simulink model "SF045A_HwAgSysArbn"  (R2013b)
settings: Solver=FixedStepDiscrete  SolverMode=SingleTasking  StartTime=0.0  StopTime=1  FixedStep=.002  RelTol=1e-3
values from neighbouring files (symbols this model uses):
  ARCHGLBPRM_2MILLISEC_SEC_F32 = DataDict.Constant    [SF045A_HwAgSysArbn_DataDict.m]
  CNVSECTOCNT_CNTPERSEC_U32 = DataDict.Constant    [SF045A_HwAgSysArbn_DataDict.m]
  CNVTOMILLISEC_MILLISECPERCNT_F32 = DataDict.Constant    [SF045A_HwAgSysArbn_DataDict.m]
  FltInj_f32 = DataDict.Client    [SF045A_HwAgSysArbn_DataDict.m]
  FLTINJ_HWAGSYSARBN_HWAG = DataDict.Constant    [SF045A_HwAgSysArbn_DataDict.m]
  FLTINJ_HWAGSYSARBN_SERLCOMHWAG = DataDict.Constant    [SF045A_HwAgSysArbn_DataDict.m]
  HwAgSysArbnHwAgConf1Snsr = DataDict.Calibration    [SF045A_HwAgSysArbn_DataDict.m]
  HwAgSysArbnHwAgConf2Snsr = DataDict.Calibration    [SF045A_HwAgSysArbn_DataDict.m]
  HwAgSysArbnHwAgConfNoSnsr = DataDict.Calibration    [SF045A_HwAgSysArbn_DataDict.m]
  HwAgSysArbnHwAgCorrdCorrlnThd = DataDict.Calibration    [SF045A_HwAgSysArbn_DataDict.m]
  HwAgSysArbnHwAgCorrlnFailDebStep = DataDict.Calibration    [SF045A_HwAgSysArbn_DataDict.m]
  HwAgSysArbnHwAgCorrlnPassDebStep = DataDict.Calibration    [SF045A_HwAgSysArbn_DataDict.m]
  HwAgSysArbnHwAgCorrlnRng = DataDict.Calibration    [SF045A_HwAgSysArbn_DataDict.m]
  HwAgSysArbnHwAgSlewRate = DataDict.Calibration    [SF045A_HwAgSysArbn_DataDict.m]
  HwAgSysArbnHwAgSnsrlsCorrlnThd = DataDict.Calibration    [SF045A_HwAgSysArbn_DataDict.m]
  HwAgSysArbnHwAgSnsrlsKineThd = DataDict.Calibration    [SF045A_HwAgSysArbn_DataDict.m]
  HwAgSysArbnHwAgToMotAgCorrlnElpdTiLim = DataDict.Calibration    [SF045A_HwAgSysArbn_DataDict.m]
  HwAgSysArbnSerlComHwAgCorrdConf = DataDict.Calibration    [SF045A_HwAgSysArbn_DataDict.m]
  HwAgSysArbnSerlComHwAgSnsrlsConf = DataDict.Calibration    [SF045A_HwAgSysArbn_DataDict.m]
  HwAgSysArbnSlewRateTmr = DataDict.Calibration    [SF045A_HwAgSysArbn_DataDict.m]
  HWAGTHD_ULS_FLOAT32 = DataDict.Constant    [SF045A_HwAgSysArbn_DataDict.m]
  INVLDSRC_CNT_S08 = DataDict.Constant    [SF045A_HwAgSysArbn_DataDict.m]
  LRGSLEW_HWDEGPERSEC_F32 = DataDict.Constant    [SF045A_HwAgSysArbn_DataDict.m]
  NODEBSTEP_CNT_U16 = DataDict.Constant    [SF045A_HwAgSysArbn_DataDict.m]
  SLEWINPROGS_CNT_LGC = DataDict.Constant    [SF045A_HwAgSysArbn_DataDict.m]
  SLEWNOTINPROGS_CNT_LGC = DataDict.Constant    [SF045A_HwAgSysArbn_DataDict.m]
  SNSRDATASRCSELD_CNT_S08 = DataDict.Constant    [SF045A_HwAgSysArbn_DataDict.m]
  SNSRLSDATASRCSELD_CNT_S08 = DataDict.Constant    [SF045A_HwAgSysArbn_DataDict.m]
  ZEROTMR_MILLISEC_F32 = DataDict.Constant    [SF045A_HwAgSysArbn_DataDict.m]
undefined symbols (not defined in the file or in its folder): NtcNr1, NtcSts1
libraries: simulink x10, NxtrLim x7, autosarlib x2, NxtrAbslt x2
(part 1 of 3)
settings Model: PauseTimes=0.48  CovFilter=UTP_SF045A_HwAgSysArbn_cov_flt_list  CovHTMLOptions=-sRT=1 -aTS=1 -bRG=1 -bTC=1 -hTR=0 -nFC=0 -scm=1 -bcm=1 -xEv=0  Creator=TZ5743  LastModifiedBy=TZ5743
settings SolverCC: AutoInsertRateTranBlk=on  InsertRTBMode=Always
settings DataIOCC: LimitDataPoints=off  SaveFormat=Structure  ReturnWorkspaceOutputs=on
settings OptimizationCC: BlockReduction=off  InlineParams=on  ZeroExternalMemoryAtStartup=off  ZeroInternalMemoryAtStartup=off  OptimizeModelRefInitCode=on  LifeSpan=1
settings DebuggingCC: SignalInfNanChecking=error  SignalRangeChecking=warning  UnderspecifiedInitializationDetection=Simplified  SolverPrmCheckMsg=error  InheritedTsInSrcMsg=error  DiscreteInheritContinuousMsg=error  SingleTaskRateTransMsg=error  TasksWithSamePriorityMsg=error  SigSpecEnsureSampleTimeMsg=error  CheckMatrixSingularityMsg=error  ParameterUnderflowMsg=error  ParameterPrecisionLossMsg=error  ParameterTunabilityLossMsg=error  FixptConstUnderflowMsg=warning  FixptConstOverflowMsg=warning  VectorMatrixConversionMsg=error  SignalLabelMismatchMsg=error  UnconnectedInputMsg=error  UnconnectedOutputMsg=error  UnconnectedLineMsg=error  SFcnCompatibilityMsg=error  UniqueDataStoreMsg=warning  BusObjectLabelMismatch=error  RootOutportRequireBusObject=error  AssertControl=DisableAll  ModelReferenceIOMsg=error  ModelReferenceVersionMismatchMessage=warning  ModelReferenceIOMismatchMessage=error  ModelReferenceCSMismatchMessage=warning  ModelReferenceDataLoggingMessage=error  StateNameClashWarn=warning  StrictBusMsg=ErrorOnBusTreatedAsVector  NonBusSignalsTreatedAsBus=error  SFUnexpectedBacktrackingDiag=error  SFInvalidInputDataAccessInChartInitDiag=error  SFNoUnconditionalDefaultTransitionDiag=error  SFTransitionOutsideNaturalParentDiag=error  SFUnconditionalTransitionShadowingDiag=error  SFUndirectedBroadcastEventsDiag=error
settings ModelReferenceCC: ModelReferenceNumInstancesAllowed=Single
settings RTWCC: SystemTargetFile=autosar.tlc  GenCodeOnly=on  TemplateMakefile=ert_default_tmf  Description=AUTOSAR  GenerateReport=on  ProcessScript=autosar_make_rtw_hook  LaunchReport=on
settings CodeAppCC: GenerateComments=off  IgnoreCustomStorageClasses=off  CustomSymbolStrType=$N$R$M  CustomSymbolStrBlkIO=$N$M  SimulinkBlockComments=off
settings STFCustomTargetCC: ParMdlRefBuildCompliant=on  CompOptLevelCompliant=on  IncludeMdlTerminateFcn=off  CombineOutputUpdateFcns=on  SuppressErrorStatus=on  ERTFirstTimeCompliant=on  ERTCustomFileBanners=on  SupportNonFinite=off  SupportComplex=off  SupportContinuousTime=off  SupportNonInlinedSFcns=off  MATLABClassNameForMDSCustomization=Simulink.SoftwareTarget.ERTCustomization  AutosarCompliant=on  GRTInterface=off  SystemTargetFile=autosar.tlc
settings ERTTargetCC: CodeReplacementLibrary=ANSI_C  ConcurrentExecutionCompliant=off  IncludeMdlTerminateFcn=off  SuppressErrorStatus=on  SupportNonFinite=off  SupportComplex=off  ModelStepFunctionPrototypeControlCompliant=off  CPPClassGenCompliant=off  AutosarCompliant=on  InlinedParameterPlacement=NonHierarchical  ERTCustomFileTemplate=example_file_process.tlc  EnableUserReplacementTypes=on

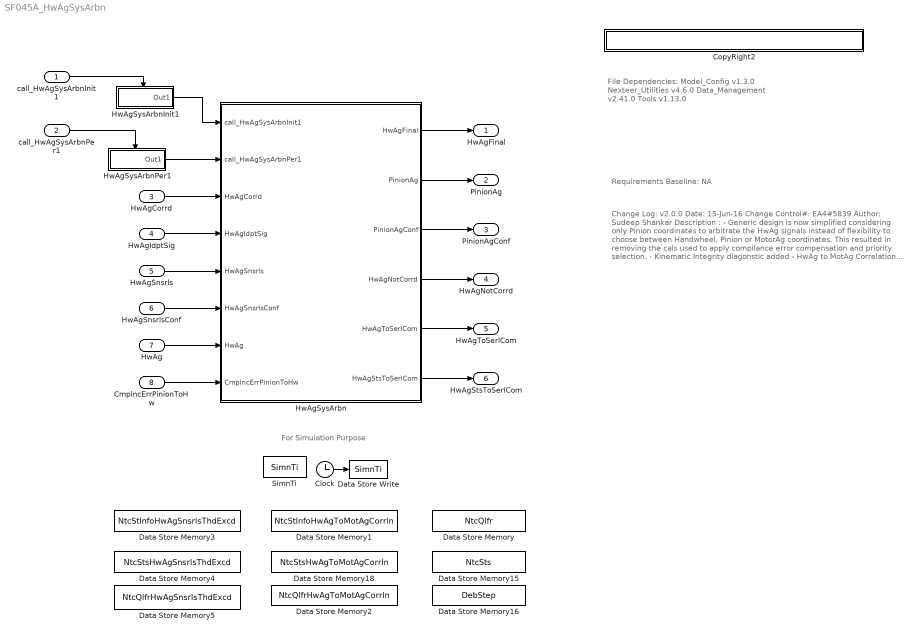
== system SF045A_HwAgSysArbn ==
  note: For Simulation Purpose
  note: File Dependencies:
      |
      | Model_Config v1.3.0
      | Nexteer_Utilities v4.6.0
      | Data_Management v2.41.0
      | Tools v1.13.0
  note: Requirements Baseline: NA
  note: Change Log:
      |
      | v2.0.0
      | Date: 15-Jun-16
      | Change Control#: EA4#5839
      | Author: Sudeep Shankar
      | Description :
      | - Generic design is now simplified considering only Pinion
      | coordinates to arbitrate the HwAg signals instead of flexibility to
      | choose between Handwheel, Pinion or MotorAg coordinates.
      | This resulted in removing the cals used to apply compilance error
      | compensation and priority selection.
      | - Kinematic Integrity diagonstic added
      | - HwAg to MotAg Correlation diagonstic added
      | - Logic added to arbitrate HwAg signal going to EOT when HwAg
      | sensor signals not available.
      |
      | v1.1.0
      | Date: 12-Sep-2015
      | Change Control #: EA4#860
      | Author:  Sudeep Shankar
      | Description:
      | - Minor modification in source change logic
      |  detection to avoid ambiguity in state variable
      |  read and write priorities
      | - Setting Initial condition of while loop to 'true'
      | instead of comparing greater than 1.
      | - Removed signal conversion blocks wherever
      | not required.
      | - Set while loop iteration to '-1' instead of restricting
      | it to '5' as condition check is in place to restrict
      | while iteration equal to number of signals present.
      |
      | v1.0.0
      | Date: 28-Aug-2015
      | Change Control #: EA4#860
      | Author:  Sudeep Shankar
      | Description:
      | - EA4 Initial Release
  call_HwAgSysArbnInit1 : Inport
  call_HwAgSysArbnPer1 : Inport  Port=2
  HwAgCorrd : Inport  RequirementInfo={} %GIDa_cc9a7bcf_75f9_45c8_a24f_b8479fae80cf  Port=3
  HwAgIdptSig : Inport  RequirementInfo={} %GIDa_9a7b919a_3c4b_44c1_bb96_545a47b8b3d3  Port=4
  HwAgSnsrls : Inport  RequirementInfo={} %GIDa_eede448f_64dd_4146_b16f_6fc16ca31f60  Port=5
  HwAgSnsrlsConf : Inport  RequirementInfo={} %GIDa_f6d9b3ed_9576_46cf_8319_2d07116884b2  Port=6
  HwAg : Inport  RequirementInfo={} %GIDa_3ab8439e_d791_45cf_9b38_dc1d6a5d96c4  Port=7
  CmplncErrPinionToHw : Inport  RequirementInfo={} %GIDa_8afc3a2b_29a0_4b25_ac8f_049b17fb3d6a  Port=8
  Clock : Clock
  CopyRight2 : Subsystem  Description=|  mask(Copyright Information){none=on}
      | Copyright info block.                                               
      |                                                                     
      | Place copyright information at the top of every subsystem in design.
      mask prompts: none "No parameters"
      mask help: Place copyright information at the top of every subsystem in design.
      mask Display:
      | NxtrConf = 'Nexteer Confidential';
      | 
      | sys = bdroot; %handle for the current model ("system")
      | first = get_param(sys,'Created');
      | first = first(end-3:end);  %year is last four digits
      | 
      | last = get_param(sys,'LastModifiedDate');
      | if isempty(last)
      |     last = datestr(now,'yyyy');
      | else
      |     last = last(end-3:end);
      | end
      | 
      | if strcmp(first,last)
      |     fprintf('%s -- Copyright %s Nexteer',NxtrConf,first)
      | else
      |     fprintf('%s -- %s%s- %s Nexteer',NxtrConf,char(169),first,last)
      | end
  Data Store Memory : DataStoreMemory  DataStoreName=NtcQlfr  InitialValue=SigQlfr1.SIGQLFR_NORES  OutDataTypeStr=Enum: SigQlfr1
  Data Store Memory1 : DataStoreMemory  DataStoreName=NtcStInfoHwAgToMotAgCorrln  OutDataTypeStr=uint8
  Data Store Memory15 : DataStoreMemory  DataStoreName=NtcSts  InitialValue=NtcSts1.NTCSTS_PREPASSD  OutDataTypeStr=Enum: NtcSts1
  Data Store Memory16 : DataStoreMemory  DataStoreName=DebStep
  Data Store Memory18 : DataStoreMemory  DataStoreName=NtcStsHwAgToMotAgCorrln  InitialValue=NtcSts1.NTCSTS_PASSD  OutDataTypeStr=Enum: NtcSts1
  Data Store Memory2 : DataStoreMemory  DataStoreName=NtcQlfrHwAgToMotAgCorrln  InitialValue=SigQlfr1.SIGQLFR_NORES  OutDataTypeStr=Enum: SigQlfr1
  Data Store Memory3 : DataStoreMemory  DataStoreName=NtcStInfoHwAgSnsrlsThdExcd  OutDataTypeStr=uint8
  Data Store Memory4 : DataStoreMemory  DataStoreName=NtcStsHwAgSnsrlsThdExcd  InitialValue=NtcSts1.NTCSTS_PASSD  OutDataTypeStr=Enum: NtcSts1
  Data Store Memory5 : DataStoreMemory  DataStoreName=NtcQlfrHwAgSnsrlsThdExcd  InitialValue=SigQlfr1.SIGQLFR_NORES  OutDataTypeStr=Enum: SigQlfr1
  Data Store Write : DataStoreWrite  DataStoreName=SimnTi
  HwAgSysArbn : Subsystem  RequirementInfo="{}  %GIDa_b3e0ed6f_fb94_4fa4_96b1_04061689a89e"
  HwAgSysArbnInit1 : Subsystem  TreatAsAtomicUnit=on
  HwAgSysArbnPer1 : Subsystem  TreatAsAtomicUnit=on
  SimnTi : DataStoreMemory  DataStoreName=SimnTi
  HwAgFinal : Outport
  PinionAg : Outport  Port=2
  PinionAgConf : Outport  Port=3
  HwAgNotCorrd : Outport  Port=4
  HwAgToSerlCom : Outport  Port=5
  HwAgStsToSerlCom : Outport  Port=6
  wires:
  HwAgSysArbn/2(PinionAg) -> PinionAg/1
  HwAgSysArbn/3(PinionAgConf) -> PinionAgConf/1
  HwAgSysArbn/4(HwAgNotCorrd) -> HwAgNotCorrd/1
  HwAgSysArbn/1(HwAgFinal) -> HwAgFinal/1
  HwAgSysArbn/6(HwAgStsToSerlCom) -> HwAgStsToSerlCom/1
  Clock/1 -> Data Store Write/1
  HwAgSysArbn/5(HwAgToSerlCom) -> HwAgToSerlCom/1
  HwAgSysArbnInit1/1(Out1) -> HwAgSysArbn/1(call_HwAgSysArbnInit1)
  HwAgSysArbnPer1/1(Out1) -> HwAgSysArbn/2(call_HwAgSysArbnPer1)
  HwAgSnsrls/1 -> HwAgSysArbn/5(HwAgSnsrls)
  HwAgCorrd/1 -> HwAgSysArbn/3(HwAgCorrd)
  HwAgSnsrlsConf/1 -> HwAgSysArbn/6(HwAgSnsrlsConf)
  HwAgIdptSig/1 -> HwAgSysArbn/4(HwAgIdptSig)
  CmplncErrPinionToHw/1 -> HwAgSysArbn/8(CmplncErrPinionToHw)
  HwAg/1 -> HwAgSysArbn/7(HwAg)
  call_HwAgSysArbnInit1/1 -> HwAgSysArbnInit1/Enable
  call_HwAgSysArbnPer1/1 -> HwAgSysArbnPer1/Enable

== system SF045A_HwAgSysArbn/CopyRight2 ==

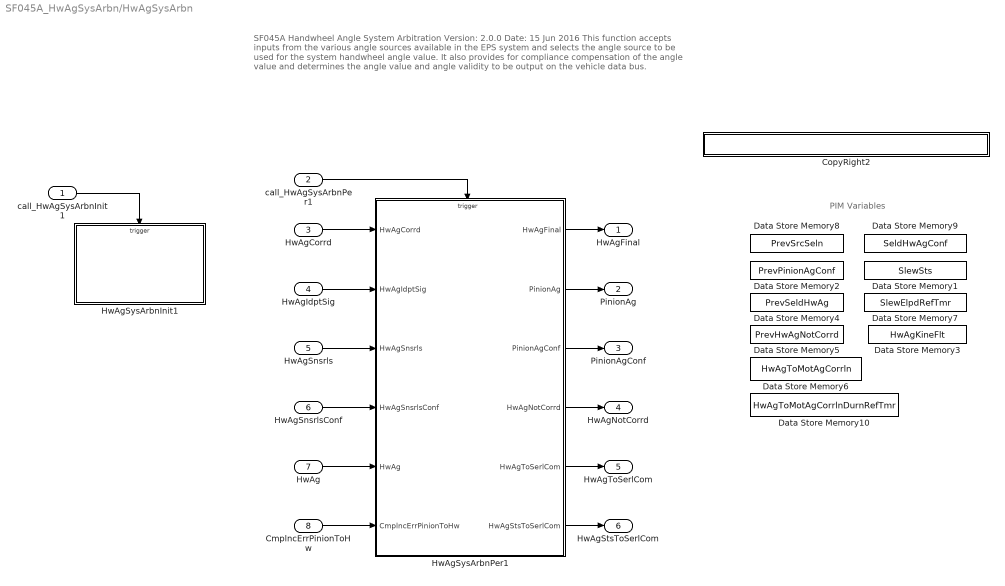
== system SF045A_HwAgSysArbn/HwAgSysArbn ==
  note: PIM Variables
  note: SF045A  Handwheel Angle System Arbitration       Version: 2.0.0                                                        Date: 15 Jun 2016
      |
      | This function accepts inputs from the various angle sources available in the EPS system and selects the angle
      | source to be used for the system handwheel angle value. It also provides for compliance compensation of the
      | angle value and determines the angle value and angle validity to be output on the vehicle data bus.
  call_HwAgSysArbnInit1 : Inport
  call_HwAgSysArbnPer1 : Inport  Port=2
  HwAgCorrd : Inport  RequirementInfo={} %GIDa_0c48395d_f55e_4aa8_967c_ddfcd5dc0f09  Port=3
  HwAgIdptSig : Inport  RequirementInfo={} %GIDa_050c3700_87b8_4e6a_a603_fe10bf5bb98d  Port=4
  HwAgSnsrls : Inport  RequirementInfo={} %GIDa_2af70a6d_5cf9_42e5_985f_0de67760f974  Port=5
  HwAgSnsrlsConf : Inport  RequirementInfo={} %GIDa_205f4441_a425_4e75_91eb_166c28519f31  Port=6
  HwAg : Inport  RequirementInfo={} %GIDa_bd860903_e40a_4856_a107_6e65debfd627  Port=7
  CmplncErrPinionToHw : Inport  RequirementInfo={} %GIDa_fd50d5ef_7c8c_43a4_8956_a275e6267051  Port=8
  CopyRight2 : Subsystem  Description=|  mask(Copyright Information){none=on}
      | Copyright info block.                                               
      |                                                                     
      | Place copyright information at the top of every subsystem in design.
      mask prompts: none "No parameters"
      mask help: Place copyright information at the top of every subsystem in design.
      mask Display:
      | NxtrConf = 'Nexteer Confidential';
      | 
      | sys = bdroot; %handle for the current model ("system")
      | first = get_param(sys,'Created');
      | first = first(end-3:end);  %year is last four digits
      | 
      | last = get_param(sys,'LastModifiedDate');
      | if isempty(last)
      |     last = datestr(now,'yyyy');
      | else
      |     last = last(end-3:end);
      | end
      | 
      | if strcmp(first,last)
      |     fprintf('%s -- Copyright %s Nexteer',NxtrConf,first)
      | else
      |     fprintf('%s -- %s%s- %s Nexteer',NxtrConf,char(169),first,last)
      | end
  Data Store Memory1 : DataStoreMemory  DataStoreName=SlewSts  StateMustResolveToSignalObject=on
  Data Store Memory10 : DataStoreMemory  DataStoreName=HwAgToMotAgCorrlnDurnRefTmr  StateMustResolveToSignalObject=on
  Data Store Memory2 : DataStoreMemory  DataStoreName=PrevPinionAgConf  StateMustResolveToSignalObject=on
  Data Store Memory3 : DataStoreMemory  DataStoreName=HwAgKineFlt  StateMustResolveToSignalObject=on
  Data Store Memory4 : DataStoreMemory  DataStoreName=PrevSeldHwAg  StateMustResolveToSignalObject=on
  Data Store Memory5 : DataStoreMemory  DataStoreName=PrevHwAgNotCorrd  StateMustResolveToSignalObject=on
  Data Store Memory6 : DataStoreMemory  DataStoreName=HwAgToMotAgCorrln  StateMustResolveToSignalObject=on
  Data Store Memory7 : DataStoreMemory  DataStoreName=SlewElpdRefTmr  StateMustResolveToSignalObject=on
  Data Store Memory8 : DataStoreMemory  DataStoreName=PrevSrcSeln  StateMustResolveToSignalObject=on
  Data Store Memory9 : DataStoreMemory  DataStoreName=SeldHwAgConf  StateMustResolveToSignalObject=on
  HwAgSysArbnInit1 : Subsystem  TreatAsAtomicUnit=on
  HwAgSysArbnPer1 : Subsystem
  HwAgFinal : Outport  RequirementInfo={} %GIDa_011fe0ec_bcc0_4a9e_bfa8_b93370ffdc5f
  PinionAg : Outport  RequirementInfo={} %GIDa_f176d339_cae7_40f0_af7d_2598900e3a6e  Port=2
  PinionAgConf : Outport  RequirementInfo={} %GIDa_ba6f2b72_e674_40ee_820e_69cfc9bdaacd  Port=3
  HwAgNotCorrd : Outport  RequirementInfo={} %GIDa_667dfd31_56c6_4848_b6a8_5a3d7a5632fb  Port=4
  HwAgToSerlCom : Outport  RequirementInfo={} %GIDa_8096249c_a6e2_4a31_b51a_c06af36d6bde  Port=5
  HwAgStsToSerlCom : Outport  RequirementInfo={} %GIDa_30b9e9dd_ad37_434a_8538_15d621b4541c  Port=6
  wires:
  call_HwAgSysArbnPer1/1 -> HwAgSysArbnPer1/Trigger
  call_HwAgSysArbnInit1/1 -> HwAgSysArbnInit1/Trigger
  HwAgSysArbnPer1/4(HwAgNotCorrd) -> HwAgNotCorrd/1
  HwAgSysArbnPer1/2(PinionAg) -> PinionAg/1
  HwAgSysArbnPer1/6(HwAgStsToSerlCom) -> HwAgStsToSerlCom/1
  HwAgSysArbnPer1/5(HwAgToSerlCom) -> HwAgToSerlCom/1
  HwAgSysArbnPer1/3(PinionAgConf) -> PinionAgConf/1
  HwAgSnsrls/1 -> HwAgSysArbnPer1/3(HwAgSnsrls)
  HwAgCorrd/1 -> HwAgSysArbnPer1/1(HwAgCorrd)
  HwAgSnsrlsConf/1 -> HwAgSysArbnPer1/4(HwAgSnsrlsConf)
  HwAgIdptSig/1 -> HwAgSysArbnPer1/2(HwAgIdptSig)
  CmplncErrPinionToHw/1 -> HwAgSysArbnPer1/6(CmplncErrPinionToHw)
  HwAg/1 -> HwAgSysArbnPer1/5(HwAg)
  HwAgSysArbnPer1/1(HwAgFinal) -> HwAgFinal/1

== system SF045A_HwAgSysArbn/HwAgSysArbnInit1 ==
  Enable : EnablePort
  Function-Call Generator : simulink/Ports & Subsystems/Function-Call Generator  sample_time=.002  numberOfIterations=1
  Out1 : Outport
  wires:
  Function-Call Generator/1 -> Out1/1

== system SF045A_HwAgSysArbn/HwAgSysArbnPer1 ==
  Enable : EnablePort
  call_HwAgSysArbnPer1 : simulink/Ports & Subsystems/Function-Call Generator  RequirementInfo={} %GIDa_ec825fb2_121b_4b6b_b290_bf31fce876d3  sample_time=0.002  numberOfIterations=1
  Out1 : Outport
  wires:
  call_HwAgSysArbnPer1/1 -> Out1/1

== system SF045A_HwAgSysArbn/HwAgSysArbn/CopyRight2 ==

== system SF045A_HwAgSysArbn/HwAgSysArbn/HwAgSysArbnInit1 ==
  note: Set Kinematic Integrity Diagostic to PASS
  note: 'PrevSrcSeln' is set to "INVALID SOURCE" in initialization to ensure that source change is detected
      | when source selection happens for the first time after initialization.
  note: Initialize Slew State to "Not in progress" at startup
  function : TriggerPort  TriggerType=function-call
  Constant1 : Constant  RequirementInfo={} %GIDa_bd6cf35a_c752_43ca_93be_9c9b276a6240  Value=0
  Constant2 : Constant  RequirementInfo={} %GIDa_50809f46_4379_44ea_9224_8e996deda18f  Value=NODEBSTEP_CNT_U16
  Constant7 : Constant  Value=SLEWNOTINPROGS_CNT_LGC
  CopyRight2 : Subsystem  Description=|  mask(Copyright Information){none=on}
      | Copyright info block.                                               
      |                                                                     
      | Place copyright information at the top of every subsystem in design.
      mask prompts: none "No parameters"
      mask help: Place copyright information at the top of every subsystem in design.
      mask Display:
      | NxtrConf = 'Nexteer Confidential';
      | 
      | sys = bdroot; %handle for the current model ("system")
      | first = get_param(sys,'Created');
      | first = first(end-3:end);  %year is last four digits
      | 
      | last = get_param(sys,'LastModifiedDate');
      | if isempty(last)
      |     last = datestr(now,'yyyy');
      | else
      |     last = last(end-3:end);
      | end
      | 
      | if strcmp(first,last)
      |     fprintf('%s -- Copyright %s Nexteer',NxtrConf,first)
      | else
      |     fprintf('%s -- %s%s- %s Nexteer',NxtrConf,char(169),first,last)
      | end
  Data Store Write1 : DataStoreWrite  RequirementInfo={} %GIDa_ed78b567_a6b6_41da_bf60_9df352ceaf90  DataStoreName=HwAgToMotAgCorrlnDurnRefTmr
  Data Store Write5 : DataStoreWrite  RequirementInfo={} %GIDa_5976233f_3450_4a81_8e0a_eaaf4d56a88e  DataStoreName=SlewSts
  Data Store Write6 : DataStoreWrite  RequirementInfo={} %GIDa_4cb2551e_dfbf_4575_8209_178b050baa05  DataStoreName=PrevSrcSeln
  Enumerated Constant1 : simulink/Sources/Enumerated Constant  RequirementInfo={} %GIDa_78dbafe2_a67d_4f00_b984_ee6afb604272  OutDataTypeStr=Enum: NtcSts1  Value=NtcSts1.NTCSTS_PASSD  SampleTime=inf
  Enumerated Constant2 : simulink/Sources/Enumerated Constant  RequirementInfo={} %GIDa_10ca5e51_019d_4f39_90cb_2775e488d2b0  OutDataTypeStr=Enum: NtcNr1  Value=NtcNr1.NTCNR_0X0A1  SampleTime=inf
  GetRefTmr100MicroSec32bit : Subsystem  RequirementInfo={} %GIDa_f5914e2f_3dac_4251_b655_ba1168612562
  Kinematic Integrity : Subsystem  RequirementInfo={} %GIDa_e2a8d71c_6639_4a30_b92d_fbf0b44b7e0b  mask(SetNTC){}
      mask help: SetNTC library block
  SET1 : Constant  RequirementInfo={} %GIDa_173d0037_1d29_4d18_8e95_d80bd9f8e211  Value=INVLDSRC_CNT_S08
  wires:
  Constant7/1 -> Data Store Write5/1
  SET1/1 -> Data Store Write6/1
  Enumerated Constant1/1 -> Kinematic Integrity/3(NtcSts)
  Constant1/1 -> Kinematic Integrity/2(NtcStInfo)
  Enumerated Constant2/1 -> Kinematic Integrity/1(NtcNr)
  Constant2/1 -> Kinematic Integrity/4(DebStep)
  GetRefTmr100MicroSec32bit/1(RefTmr) -> Data Store Write1/1

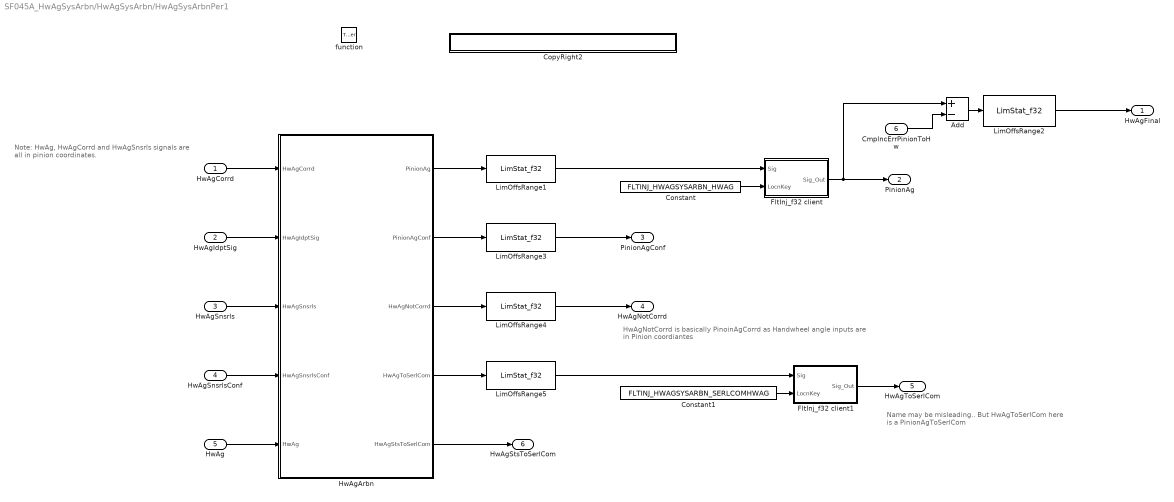
== system SF045A_HwAgSysArbn/HwAgSysArbn/HwAgSysArbnPer1 ==
  note: Name may be misleading..
      | But HwAgToSerlCom here is a PinionAgToSerlCom
  note: HwAgNotCorrd is basically PinoinAgCorrd as Handwheel angle inputs
      | are in Pinion coordiantes
  note: Note: HwAg, HwAgCorrd and HwAgSnsrls signals
      | are all in pinion coordinates.
  HwAgCorrd : Inport
  HwAgIdptSig : Inport  Port=2
  HwAgSnsrls : Inport  Port=3
  HwAgSnsrlsConf : Inport  Port=4
  HwAg : Inport  Port=5
  CmplncErrPinionToHw : Inport  Port=6
  function : TriggerPort  TriggerType=function-call
  Add : Sum  RequirementInfo={} %GIDa_c649b52e_fa89_4806_ad65_f5109016dce6  Inputs=+-
  Constant : Constant  Value=FLTINJ_HWAGSYSARBN_HWAG
  Constant1 : Constant  Value=FLTINJ_HWAGSYSARBN_SERLCOMHWAG
  CopyRight2 : Subsystem  Description=|  mask(Copyright Information){none=on}
      | Copyright info block.                                               
      |                                                                     
      | Place copyright information at the top of every subsystem in design.
      mask prompts: none "No parameters"
      mask help: Place copyright information at the top of every subsystem in design.
      mask Display:
      | NxtrConf = 'Nexteer Confidential';
      | 
      | sys = bdroot; %handle for the current model ("system")
      | first = get_param(sys,'Created');
      | first = first(end-3:end);  %year is last four digits
      | 
      | last = get_param(sys,'LastModifiedDate');
      | if isempty(last)
      |     last = datestr(now,'yyyy');
      | else
      |     last = last(end-3:end);
      | end
      | 
      | if strcmp(first,last)
      |     fprintf('%s -- Copyright %s Nexteer',NxtrConf,first)
      | else
      |     fprintf('%s -- %s%s- %s Nexteer',NxtrConf,char(169),first,last)
      | end
  FltInj_f32 client : Subsystem  RequirementInfo={} %GIDa_92f81fd3_ecd2_4636_a4d0_e916ab63c8f1  Variant=on
      settings: GeneratePreprocessorConditionals=on
  FltInj_f32 client1 : Subsystem  RequirementInfo={} %GIDa_e87011ff_af47_4e76_bd4f_a2053c2ac98e  Variant=on
      settings: GeneratePreprocessorConditionals=on
  HwAgArbn : Subsystem
  LimOffsRange{1..2,4..5} (4 alike) : NxtrLim/LimStat_f32  LoLim=PINIONAGLOWLIM_HWDEG_F32  HiLim=PINIONAGHILIM_HWDEG_F32
      settings: AttributesFormatString=|
      | Low Limit: %<LoLim>
      | High Limit:%<HiLim>
  LimOffsRange3 : NxtrLim/LimStat_f32  LoLim=PINIONAGCONFLOWLIM_ULS_F32  HiLim=PINIONAGCONFHILIM_ULS_F32
      settings: AttributesFormatString=|
      | Low Limit: %<LoLim>
      | High Limit:%<HiLim>
  HwAgFinal : Outport
  PinionAg : Outport  Port=2
  PinionAgConf : Outport  Port=3
  HwAgNotCorrd : Outport  Port=4
  HwAgToSerlCom : Outport  Port=5
  HwAgStsToSerlCom : Outport  Port=6
  wires:
  LimOffsRange3/1 -> PinionAgConf/1
  Add/1 -> LimOffsRange2/1
  LimOffsRange1/1 -> FltInj_f32 client/1(Sig)
  Constant/1 -> FltInj_f32 client/2("LocnKey  ")
  LimOffsRange5/1 -> FltInj_f32 client1/1(Sig)
  FltInj_f32 client1/1(Sig_Out) -> HwAgToSerlCom/1
  Constant1/1 -> FltInj_f32 client1/2("LocnKey  ")
  FltInj_f32 client/1(Sig_Out) -> PinionAg/1, Add/1
  LimOffsRange4/1 -> HwAgNotCorrd/1
  HwAgSnsrlsConf/1 -> HwAgArbn/4(HwAgSnsrlsConf)
  HwAgIdptSig/1 -> HwAgArbn/2(HwAgIdptSig)
  CmplncErrPinionToHw/1 -> Add/2
  LimOffsRange2/1 -> HwAgFinal/1
  HwAgSnsrls/1 -> HwAgArbn/3(HwAgSnsrls)
  HwAg/1 -> HwAgArbn/5(HwAg)
  HwAgArbn/1(PinionAg) -> LimOffsRange1/1
  HwAgArbn/2(PinionAgConf) -> LimOffsRange3/1
  HwAgArbn/4(HwAgToSerlCom) -> LimOffsRange5/1
  HwAgArbn/5(HwAgStsToSerlCom) -> HwAgStsToSerlCom/1
  HwAgArbn/3(HwAgNotCorrd) -> LimOffsRange4/1
  HwAgCorrd/1 -> HwAgArbn/1(HwAgCorrd)

== system SF045A_HwAgSysArbn/HwAgSysArbn/HwAgSysArbnInit1/CopyRight2 ==

== system SF045A_HwAgSysArbn/HwAgSysArbn/HwAgSysArbnInit1/GetRefTmr100MicroSec32bit ==
  note: 1 count = 100 uSec
  note: seconds
  note: microseconds
  note: counts
  note: Wrap-to-zero
  note: GetRefTmr100MicroSec32bit
  CopyRight2 : Subsystem  Description=|  mask(Copyright Information){none=on}
      | Copyright info block.                                               
      |                                                                     
      | Place copyright information at the top of every subsystem in design.
      mask prompts: none "No parameters"
      mask help: Place copyright information at the top of every subsystem in design.
      mask Display:
      | NxtrConf = 'Nexteer Confidential';
      | 
      | sys = bdroot; %handle for the current model ("system")
      | first = get_param(sys,'Created');
      | if(isempty(first))
      |     first = datestr(now,'yyyy');
      | else
      |     first = first(end-3:end);  %year is last four digits
      | end
      | 
      | last = get_param(sys,'LastModifiedDate');
      | if isempty(last)
      |     last = datestr(now,'yyyy');
      | else
      |     last = last(end-3:end);
      | end
      | 
      | if strcmp(first,last)
      |     fprintf('%s -- Copyright %s Nexteer',NxtrConf,first)
      | else
      |     fprintf('%s -- %s%s- %s Nexteer',NxtrConf,char(169),first,last)
      | end
  Count per uSec : Constant  Value=0.01
  Data Store Read1 : DataStoreRead  DataStoreName=SimnTi
  Data Type Conversion1 : DataTypeConversion  OutDataTypeStr=uint32
  Divide1 : Product  Inputs=**
  Divide2 : Product  Inputs=*/
  Max Counts : Constant  Value=2^32-1
  Product1 : Product
  Product2 : Product
  Rounding : Rounding
  Subtract1 : Sum  Inputs=+-
  uSec per Sec : Constant  Value=1000000
  RefTmr : Outport
  wires:
  Product2/1 -> Subtract1/2
  Subtract1/1 -> Data Type Conversion1/1
  Rounding/1 -> Product2/1
  Divide2/1 -> Rounding/1
  Max Counts/1 -> Divide2/2, Product2/2
  Divide1/1 -> Divide2/1, Subtract1/1
  Product1/1 -> Divide1/1
  Data Store Read1/1 -> Product1/1
  Count per uSec/1 -> Divide1/2
  uSec per Sec/1 -> Product1/2
  Data Type Conversion1/1 -> RefTmr/1

== system SF045A_HwAgSysArbn/HwAgSysArbn/HwAgSysArbnInit1/Kinematic Integrity ==
  NtcNr : Inport
  NtcStInfo : Inport  Port=2
  NtcSts : Inport  Port=3
  DebStep : Inport  Port=4
  SetNtcSts : Subsystem  RequirementInfo={} %GIDa_16f23167_f05b_46c3_9fcc_0dcafd7bcf3c  TreatAsAtomicUnit=on
      settings: RTWSystemCode=Inline
  wires:
  NtcStInfo/1 -> SetNtcSts/2(NtcStInfo)
  DebStep/1 -> SetNtcSts/4(DebStep)
  NtcSts/1 -> SetNtcSts/3(NtcSts)
  NtcNr/1 -> SetNtcSts/1(NtcNr)  "NtcNr"

== system SF045A_HwAgSysArbn/HwAgSysArbn/HwAgSysArbnPer1/CopyRight2 ==

== system SF045A_HwAgSysArbn/HwAgSysArbn/HwAgSysArbnPer1/FltInj_f32 client ==
  note: FltInj_f32
  note: 1) Only subsystems can be added as variant choices at this level
      | 2) Blocks cannot be connected at this level as connectivity is
      | automatically determined at simulation, based on the active variant
  note: Created Aug 18, 2015
      | Kevin Derry
  Sig : Inport  OutDataTypeStr=single
  "LocnKey  " : Inport  Port=2  OutDataTypeStr=uint16
  CodeGen : Subsystem  VariantControl=FLTINJENA == STD_ON
  CopyRight1 : Subsystem  Description=|  mask(Copyright Information){none=on}
      | Copyright info block.                                               
      |                                                                     
      | Place copyright information at the top of every subsystem in design.
      mask prompts: none "No parameters"
      mask help: Place copyright information at the top of every subsystem in design.
      mask Display:
      | NxtrConf = 'Nexteer Confidential';
      | 
      | sys = bdroot; %handle for the current model ("system")
      | first = get_param(sys,'Created');
      | if(isempty(first))
      |     first = datestr(now,'yyyy');
      | else
      |     first = first(end-3:end);  %year is last four digits
      | end
      | 
      | last = get_param(sys,'LastModifiedDate');
      | if isempty(last)
      |     last = datestr(now,'yyyy');
      | else
      |     last = last(end-3:end);
      | end
      | 
      | if strcmp(first,last)
      |     fprintf('%s -- Copyright %s Nexteer',NxtrConf,first)
      | else
      |     fprintf('%s -- %s%s- %s Nexteer',NxtrConf,char(169),first,last)
      | end
  Sim : Subsystem  TreatAsAtomicUnit=on  VariantControl=FLTINJENA ~= STD_ON  mask(Fault_Injection){}
      mask help: Simulation mode is just a pass-thru.
  Sig_Out : Outport  OutDataTypeStr=single

== system SF045A_HwAgSysArbn/HwAgSysArbn/HwAgSysArbnPer1/FltInj_f32 client1 ==
  note: Created Aug 18, 2015
      | Kevin Derry
  note: 1) Only subsystems can be added as variant choices at this level
      | 2) Blocks cannot be connected at this level as connectivity is
      | automatically determined at simulation, based on the active variant
  note: FltInj_f32
  Sig : Inport  OutDataTypeStr=single
  "LocnKey  " : Inport  Port=2  OutDataTypeStr=uint16
  CodeGen : Subsystem  VariantControl=FLTINJENA == STD_ON
  CopyRight1 : Subsystem  Description=|  mask(Copyright Information){none=on}
      | Copyright info block.                                               
      |                                                                     
      | Place copyright information at the top of every subsystem in design.
      mask prompts: none "No parameters"
      mask help: Place copyright information at the top of every subsystem in design.
      mask Display:
      | NxtrConf = 'Nexteer Confidential';
      | 
      | sys = bdroot; %handle for the current model ("system")
      | first = get_param(sys,'Created');
      | if(isempty(first))
      |     first = datestr(now,'yyyy');
      | else
      |     first = first(end-3:end);  %year is last four digits
      | end
      | 
      | last = get_param(sys,'LastModifiedDate');
      | if isempty(last)
      |     last = datestr(now,'yyyy');
      | else
      |     last = last(end-3:end);
      | end
      | 
      | if strcmp(first,last)
      |     fprintf('%s -- Copyright %s Nexteer',NxtrConf,first)
      | else
      |     fprintf('%s -- %s%s- %s Nexteer',NxtrConf,char(169),first,last)
      | end
  Sim : Subsystem  TreatAsAtomicUnit=on  VariantControl=FLTINJENA ~= STD_ON  mask(Fault_Injection){}
      mask help: Simulation mode is just a pass-thru.
  Sig_Out : Outport  OutDataTypeStr=single

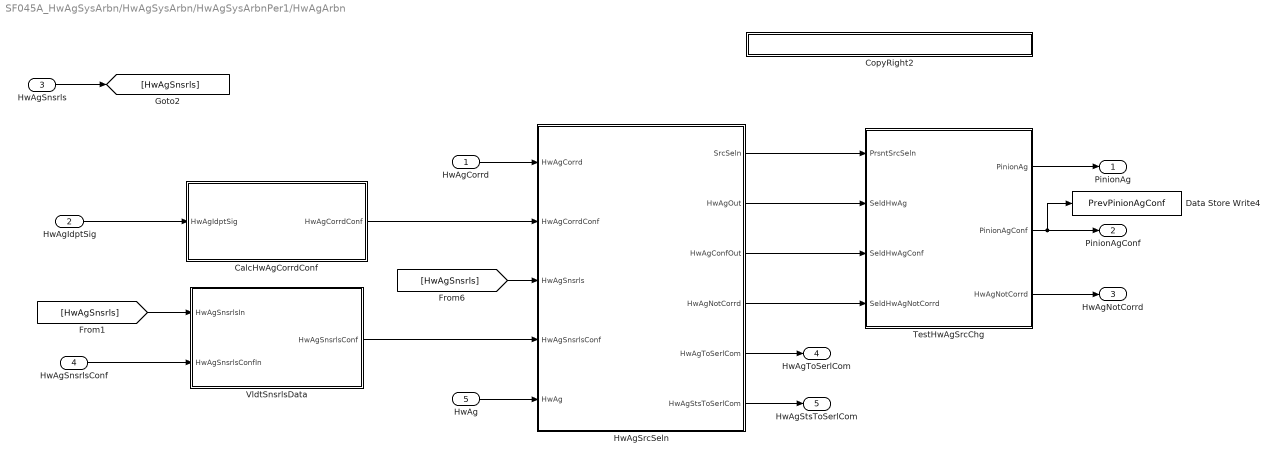
== system SF045A_HwAgSysArbn/HwAgSysArbn/HwAgSysArbnPer1/HwAgArbn ==
  HwAgCorrd : Inport
  HwAgIdptSig : Inport  Port=2
  HwAgSnsrls : Inport  Port=3
  HwAgSnsrlsConf : Inport  Port=4
  HwAg : Inport  Port=5
  "CalcHwAgCorrdConf " : Subsystem
  CopyRight2 : Subsystem  Description=|  mask(Copyright Information){none=on}
      | Copyright info block.                                               
      |                                                                     
      | Place copyright information at the top of every subsystem in design.
      mask prompts: none "No parameters"
      mask help: Place copyright information at the top of every subsystem in design.
      mask Display:
      | NxtrConf = 'Nexteer Confidential';
      | 
      | sys = bdroot; %handle for the current model ("system")
      | first = get_param(sys,'Created');
      | first = first(end-3:end);  %year is last four digits
      | 
      | last = get_param(sys,'LastModifiedDate');
      | if isempty(last)
      |     last = datestr(now,'yyyy');
      | else
      |     last = last(end-3:end);
      | end
      | 
      | if strcmp(first,last)
      |     fprintf('%s -- Copyright %s Nexteer',NxtrConf,first)
      | else
      |     fprintf('%s -- %s%s- %s Nexteer',NxtrConf,char(169),first,last)
      | end
  Data Store Write4 : DataStoreWrite  RequirementInfo={} %GIDa_b9febeb4_a0de_4de9_bb83_167b49937f1b  DataStoreName=PrevPinionAgConf
  HwAgSrcSeln : Subsystem
  TestHwAgSrcChg : Subsystem
  VldtSnsrlsData : Subsystem
  PinionAg : Outport
  PinionAgConf : Outport  Port=2
  HwAgNotCorrd : Outport  Port=3
  HwAgToSerlCom : Outport  Port=4
  HwAgStsToSerlCom : Outport  Port=5
  wires:
  HwAg/1 -> HwAgSrcSeln/5(HwAg)
  HwAgSrcSeln/1(SrcSeln) -> TestHwAgSrcChg/1(PrsntSrcSeln)
  HwAgSrcSeln/2(HwAgOut) -> TestHwAgSrcChg/2(SeldHwAg)
  HwAgSrcSeln/3(HwAgConfOut) -> TestHwAgSrcChg/3(SeldHwAgConf)
  HwAgSrcSeln/4(HwAgNotCorrd) -> TestHwAgSrcChg/4(SeldHwAgNotCorrd)
  TestHwAgSrcChg/1(PinionAg) -> PinionAg/1
  TestHwAgSrcChg/3(HwAgNotCorrd) -> HwAgNotCorrd/1
  [HwAgSnsrls] -> HwAgSrcSeln/3(HwAgSnsrls)
  HwAgSnsrlsConf/1 -> VldtSnsrlsData/2(HwAgSnsrlsConfIn)
  HwAgSnsrls/1 -> [HwAgSnsrls]
  HwAgCorrd/1 -> HwAgSrcSeln/1(HwAgCorrd)
  VldtSnsrlsData/1(HwAgSnsrlsConf) -> HwAgSrcSeln/4(HwAgSnsrlsConf)
  HwAgIdptSig/1 -> "CalcHwAgCorrdConf "/1(HwAgIdptSig)
  "CalcHwAgCorrdConf "/1(HwAgCorrdConf) -> HwAgSrcSeln/2(HwAgCorrdConf)
  HwAgSrcSeln/5(HwAgToSerlCom) -> HwAgToSerlCom/1
  HwAgSrcSeln/6(HwAgStsToSerlCom) -> HwAgStsToSerlCom/1
  [HwAgSnsrls] -> VldtSnsrlsData/1(HwAgSnsrlsIn)
  TestHwAgSrcChg/2(PinionAgConf) -> Data Store Write4/1, PinionAgConf/1

== system SF045A_HwAgSysArbn/HwAgSysArbn/HwAgSysArbnInit1/GetRefTmr100MicroSec32bit/CopyRight2 ==

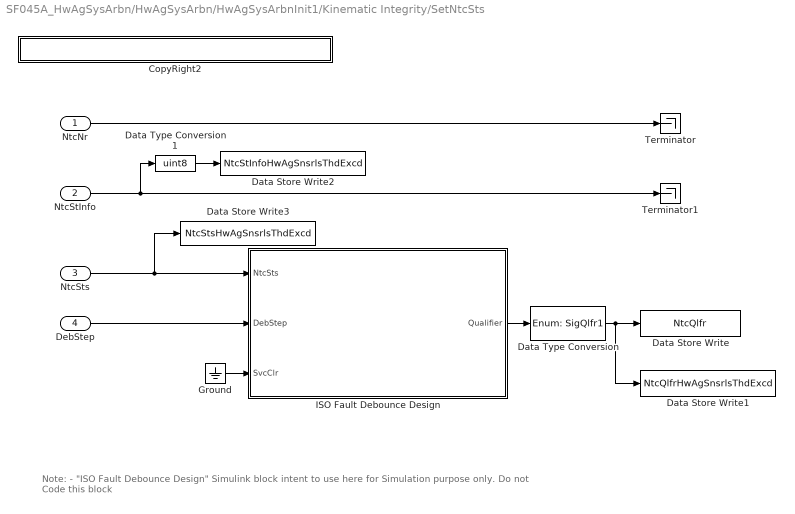
== system SF045A_HwAgSysArbn/HwAgSysArbn/HwAgSysArbnInit1/Kinematic Integrity/SetNtcSts ==
  note: Note:
      |
      | - "ISO Fault Debounce Design" Simulink block intent to use here for Simulation purpose only. Do not Code this block
  NtcNr : Inport
  NtcStInfo : Inport  Port=2
  NtcSts : Inport  Port=3
  DebStep : Inport  Port=4
  CopyRight2 : Subsystem  Description=|  mask(Copyright Information){none=on}
      | Copyright info block.                                               
      |                                                                     
      | Place copyright information at the top of every subsystem in design.
      mask prompts: none "No parameters"
      mask help: Place copyright information at the top of every subsystem in design.
      mask Display:
      | NxtrConf = 'Nexteer Confidential';
      | 
      | sys = bdroot; %handle for the current model ("system")
      | first = get_param(sys,'Created');
      | if(isempty(first))
      |     first = datestr(now,'yyyy');
      | else
      |     first = first(end-3:end);  %year is last four digits
      | end
      | 
      | last = get_param(sys,'LastModifiedDate');
      | if isempty(last)
      |     last = datestr(now,'yyyy');
      | else
      |     last = last(end-3:end);
      | end
      | 
      | if strcmp(first,last)
      |     fprintf('%s -- Copyright %s Nexteer',NxtrConf,first)
      | else
      |     fprintf('%s -- %s%s- %s Nexteer',NxtrConf,char(169),first,last)
      | end
  Data Store Write : DataStoreWrite  DataStoreName=NtcQlfr
  Data Store Write1 : DataStoreWrite  DataStoreName=NtcQlfrHwAgSnsrlsThdExcd
  Data Store Write2 : DataStoreWrite  DataStoreName=NtcStInfoHwAgSnsrlsThdExcd
  Data Store Write3 : DataStoreWrite  DataStoreName=NtcStsHwAgSnsrlsThdExcd
  Data Type Conversion : DataTypeConversion  OutDataTypeStr=Enum: SigQlfr1
  Data Type Conversion1 : DataTypeConversion  OutDataTypeStr=uint8
  Ground : Ground
  ISO Fault Debounce Design : Stateflow chart  TreatAsAtomicUnit=on
      settings: AttributesFormatString=|
      | Simulation Purpose Only.
      | Do Not Code this block
      | Diagnostic Manager Owns this requirement
  Terminator : Terminator
  Terminator1 : Terminator
  wires:
  Data Type Conversion1/1 -> Data Store Write2/1
  NtcStInfo/1 -> Terminator1/1, Data Type Conversion1/1
  NtcSts/1 -> ISO Fault Debounce Design/1(NtcSts), Data Store Write3/1
  Data Type Conversion/1 -> Data Store Write/1, Data Store Write1/1
  Ground/1 -> ISO Fault Debounce Design/3(SvcClr)
  ISO Fault Debounce Design/1(Qualifier) -> Data Type Conversion/1
  DebStep/1 -> ISO Fault Debounce Design/2(DebStep)
  NtcNr/1 -> Terminator/1

== system SF045A_HwAgSysArbn/HwAgSysArbn/HwAgSysArbnPer1/FltInj_f32 client/CodeGen ==
  note: FltInj_f32(float32 *SigPah, uint16 LocnKey)
  note: NOTE 1:  Simulink 2013b cannot handle InOut arguments, so the operation
      |                 prototype inside this block is not quite right.
      |
      | NOTE 2:  Do not use this variant for simulation.  Sig_Out = zero, always.
  Sig : Inport
  "LocnKey  " : Inport  Port=2
  CopyRight1 : Subsystem  Description=|  mask(Copyright Information){none=on}
      | Copyright info block.                                               
      |                                                                     
      | Place copyright information at the top of every subsystem in design.
      mask prompts: none "No parameters"
      mask help: Place copyright information at the top of every subsystem in design.
      mask Display:
      | NxtrConf = 'Nexteer Confidential';
      | 
      | sys = bdroot; %handle for the current model ("system")
      | first = get_param(sys,'Created');
      | if(isempty(first))
      |     first = datestr(now,'yyyy');
      | else
      |     first = first(end-3:end);  %year is last four digits
      | end
      | 
      | last = get_param(sys,'LastModifiedDate');
      | if isempty(last)
      |     last = datestr(now,'yyyy');
      | else
      |     last = last(end-3:end);
      | end
      | 
      | if strcmp(first,last)
      |     fprintf('%s -- Copyright %s Nexteer',NxtrConf,first)
      | else
      |     fprintf('%s -- %s%s- %s Nexteer',NxtrConf,char(169),first,last)
      | end
  Invoke AUTOSAR Server Operation : autosarlib/Invoke AUTOSAR Server Operation  portName=FltInj_f32  operationPrototype=FltInj_f32(IN single SigPah_ArgIn, OUT single SigPah_ArgOut, IN uint16 LocnKey)  interfacePath=/AUTOSAR/Interface  serverType=Application software  showErrorStatus=off  SAMPLETIME=-1  showARPortLabels=on
  Sig_Out : Outport  OutDataTypeStr=single
  wires:
  Invoke AUTOSAR Server Operation/1 -> Sig_Out/1
  "LocnKey  "/1 -> Invoke AUTOSAR Server Operation/2
  Sig/1 -> Invoke AUTOSAR Server Operation/1

== system SF045A_HwAgSysArbn/HwAgSysArbn/HwAgSysArbnPer1/FltInj_f32 client/CopyRight1 ==

== system SF045A_HwAgSysArbn/HwAgSysArbn/HwAgSysArbnPer1/FltInj_f32 client/Sim ==
  note: EA4.x Fault Injection
  note: This block requires no modification by FDD author.
      |
      | This block does not actually simulate any fault injection.  It is simply a pass-thru.
      |
      | Input port (#2) simply terminates its signal, but we are trying to force the FDD author
      | to properly use the FltInjectionLocType enumeration in FDD model.
  Sig : Inport
  "LocnKey  " : Inport  Port=2  OutDataTypeStr=uint16
  CopyRight1 : Subsystem  Description=|  mask(Copyright Information){none=on}
      | Copyright info block.                                               
      |                                                                     
      | Place copyright information at the top of every subsystem in design.
      mask prompts: none "No parameters"
      mask help: Place copyright information at the top of every subsystem in design.
      mask Display:
      | NxtrConf = 'Nexteer Confidential';
      | 
      | sys = bdroot; %handle for the current model ("system")
      | first = get_param(sys,'Created');
      | if(isempty(first))
      |     first = datestr(now,'yyyy');
      | else
      |     first = first(end-3:end);  %year is last four digits
      | end
      | 
      | last = get_param(sys,'LastModifiedDate');
      | if isempty(last)
      |     last = datestr(now,'yyyy');
      | else
      |     last = last(end-3:end);
      | end
      | 
      | if strcmp(first,last)
      |     fprintf('%s -- Copyright %s Nexteer',NxtrConf,first)
      | else
      |     fprintf('%s -- %s%s- %s Nexteer',NxtrConf,char(169),first,last)
      | end
  Terminator : Terminator
  Sig_Out : Outport
  wires:
  "LocnKey  "/1 -> Terminator/1
  Sig/1 -> Sig_Out/1

== system SF045A_HwAgSysArbn/HwAgSysArbn/HwAgSysArbnPer1/FltInj_f32 client1/CodeGen ==
  note: NOTE 1:  Simulink 2013b cannot handle InOut arguments, so the operation
      |                 prototype inside this block is not quite right.
      |
      | NOTE 2:  Do not use this variant for simulation.  Sig_Out = zero, always.
  note: FltInj_f32(float32 *SigPah, uint16 LocnKey)
  Sig : Inport
  "LocnKey  " : Inport  Port=2
  CopyRight1 : Subsystem  Description=|  mask(Copyright Information){none=on}
      | Copyright info block.                                               
      |                                                                     
      | Place copyright information at the top of every subsystem in design.
      mask prompts: none "No parameters"
      mask help: Place copyright information at the top of every subsystem in design.
      mask Display:
      | NxtrConf = 'Nexteer Confidential';
      | 
      | sys = bdroot; %handle for the current model ("system")
      | first = get_param(sys,'Created');
      | if(isempty(first))
      |     first = datestr(now,'yyyy');
      | else
      |     first = first(end-3:end);  %year is last four digits
      | end
      | 
      | last = get_param(sys,'LastModifiedDate');
      | if isempty(last)
      |     last = datestr(now,'yyyy');
      | else
      |     last = last(end-3:end);
      | end
      | 
      | if strcmp(first,last)
      |     fprintf('%s -- Copyright %s Nexteer',NxtrConf,first)
      | else
      |     fprintf('%s -- %s%s- %s Nexteer',NxtrConf,char(169),first,last)
      | end
  Invoke AUTOSAR Server Operation : autosarlib/Invoke AUTOSAR Server Operation  portName=FltInj_f32  operationPrototype=FltInj_f32(IN single SigPah_ArgIn, OUT single SigPah_ArgOut, IN uint16 LocnKey)  interfacePath=/AUTOSAR/Interface  serverType=Application software  showErrorStatus=off  SAMPLETIME=-1  showARPortLabels=on
  Sig_Out : Outport  OutDataTypeStr=single
  wires:
  Sig/1 -> Invoke AUTOSAR Server Operation/1
  "LocnKey  "/1 -> Invoke AUTOSAR Server Operation/2
  Invoke AUTOSAR Server Operation/1 -> Sig_Out/1

== system SF045A_HwAgSysArbn/HwAgSysArbn/HwAgSysArbnPer1/FltInj_f32 client1/CopyRight1 ==

== system SF045A_HwAgSysArbn/HwAgSysArbn/HwAgSysArbnPer1/FltInj_f32 client1/Sim ==
  note: This block requires no modification by FDD author.
      |
      | This block does not actually simulate any fault injection.  It is simply a pass-thru.
      |
      | Input port (#2) simply terminates its signal, but we are trying to force the FDD author
      | to properly use the FltInjectionLocType enumeration in FDD model.
  note: EA4.x Fault Injection
  Sig : Inport
  "LocnKey  " : Inport  Port=2  OutDataTypeStr=uint16
  CopyRight1 : Subsystem  Description=|  mask(Copyright Information){none=on}
      | Copyright info block.                                               
      |                                                                     
      | Place copyright information at the top of every subsystem in design.
      mask prompts: none "No parameters"
      mask help: Place copyright information at the top of every subsystem in design.
      mask Display:
      | NxtrConf = 'Nexteer Confidential';
      | 
      | sys = bdroot; %handle for the current model ("system")
      | first = get_param(sys,'Created');
      | if(isempty(first))
      |     first = datestr(now,'yyyy');
      | else
      |     first = first(end-3:end);  %year is last four digits
      | end
      | 
      | last = get_param(sys,'LastModifiedDate');
      | if isempty(last)
      |     last = datestr(now,'yyyy');
      | else
      |     last = last(end-3:end);
      | end
      | 
      | if strcmp(first,last)
      |     fprintf('%s -- Copyright %s Nexteer',NxtrConf,first)
      | else
      |     fprintf('%s -- %s%s- %s Nexteer',NxtrConf,char(169),first,last)
      | end
  Terminator : Terminator
  Sig_Out : Outport
  wires:
  Sig/1 -> Sig_Out/1
  "LocnKey  "/1 -> Terminator/1

== system SF045A_HwAgSysArbn/HwAgSysArbn/HwAgSysArbnPer1/HwAgArbn/CalcHwAgCorrdConf  ==
  HwAgIdptSig : Inport
  CopyRight2 : Subsystem  Description=|  mask(Copyright Information){none=on}
      | Copyright info block.                                               
      |                                                                     
      | Place copyright information at the top of every subsystem in design.
      mask prompts: none "No parameters"
      mask help: Place copyright information at the top of every subsystem in design.
      mask Display:
      | NxtrConf = 'Nexteer Confidential';
      | 
      | sys = bdroot; %handle for the current model ("system")
      | first = get_param(sys,'Created');
      | first = first(end-3:end);  %year is last four digits
      | 
      | last = get_param(sys,'LastModifiedDate');
      | if isempty(last)
      |     last = datestr(now,'yyyy');
      | else
      |     last = last(end-3:end);
      | end
      | 
      | if strcmp(first,last)
      |     fprintf('%s -- Copyright %s Nexteer',NxtrConf,first)
      | else
      |     fprintf('%s -- %s%s- %s Nexteer',NxtrConf,char(169),first,last)
      | end
  Merge1 : Merge  Inputs=4
  NoSensor : Subsystem  TreatAsAtomicUnit=on
  OneSensor : Subsystem  TreatAsAtomicUnit=on
  Switch Case : SwitchCase  CaseConditions={0,1,2}
  TwoSensors : Subsystem  TreatAsAtomicUnit=on
  Zero : Subsystem  TreatAsAtomicUnit=on
  HwAgCorrdConf : Outport
  wires:
  HwAgIdptSig/1 -> Switch Case/1
  Switch Case/1 -> NoSensor/Action
  Switch Case/4 -> Zero/Action
  Merge1/1 -> HwAgCorrdConf/1
  Switch Case/3 -> TwoSensors/Action
  Switch Case/2 -> OneSensor/Action
  NoSensor/1(Out1) -> Merge1/1
  OneSensor/1(Out1) -> Merge1/2
  TwoSensors/1(Out1) -> Merge1/3
  Zero/1(Out1) -> Merge1/4

== system SF045A_HwAgSysArbn/HwAgSysArbn/HwAgSysArbnPer1/HwAgArbn/CopyRight2 ==

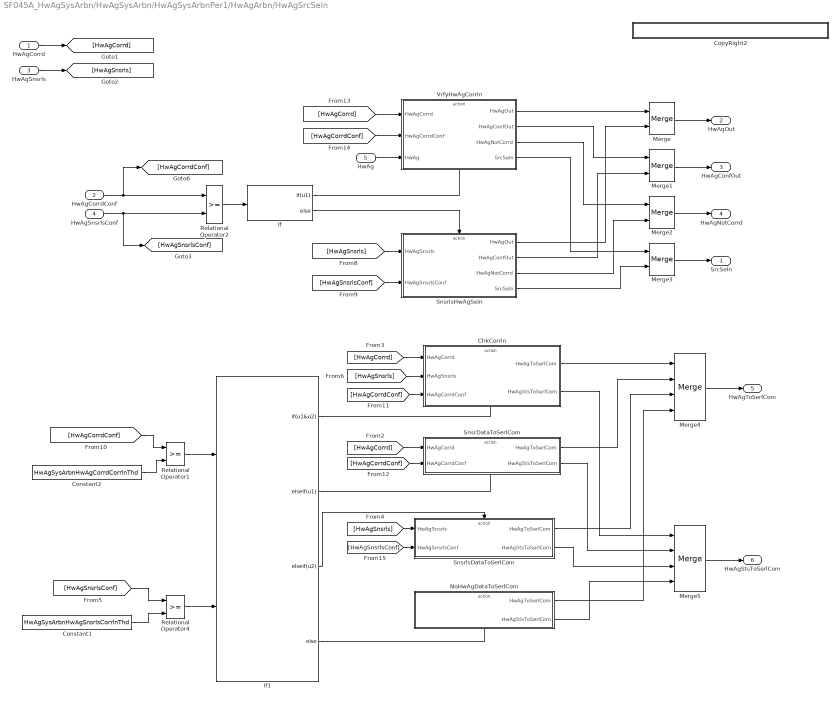
== system SF045A_HwAgSysArbn/HwAgSysArbn/HwAgSysArbnPer1/HwAgArbn/HwAgSrcSeln ==
  HwAgCorrd : Inport
  HwAgCorrdConf : Inport  Port=2
  HwAgSnsrls : Inport  Port=3
  HwAgSnsrlsConf : Inport  Port=4
  HwAg : Inport  Port=5
  ChkCorrln : Subsystem  TreatAsAtomicUnit=on
  Constant1 : Constant  RequirementInfo={} %GIDa_1e08f952_972d_4969_82e0_9bc3129f036f  Value=HwAgSysArbnHwAgSnsrlsCorrlnThd  OutDataTypeStr=single
  Constant2 : Constant  RequirementInfo={} %GIDa_99bea871_8243_4afa_9cd4_e883e34eefa7  Value=HwAgSysArbnHwAgCorrdCorrlnThd  OutDataTypeStr=single
  CopyRight2 : Subsystem  Description=|  mask(Copyright Information){none=on}
      | Copyright info block.                                               
      |                                                                     
      | Place copyright information at the top of every subsystem in design.
      mask prompts: none "No parameters"
      mask help: Place copyright information at the top of every subsystem in design.
      mask Display:
      | NxtrConf = 'Nexteer Confidential';
      | 
      | sys = bdroot; %handle for the current model ("system")
      | first = get_param(sys,'Created');
      | first = first(end-3:end);  %year is last four digits
      | 
      | last = get_param(sys,'LastModifiedDate');
      | if isempty(last)
      |     last = datestr(now,'yyyy');
      | else
      |     last = last(end-3:end);
      | end
      | 
      | if strcmp(first,last)
      |     fprintf('%s -- Copyright %s Nexteer',NxtrConf,first)
      | else
      |     fprintf('%s -- %s%s- %s Nexteer',NxtrConf,char(169),first,last)
      | end
  If : If  IfExpression=u1
  If1 : If  NumInputs=2  IfExpression=u1&u2  ElseIfExpressions=u1, u2
  Merge{,1..3} (4 alike) : Merge
  Merge4 : Merge  Inputs=4
  Merge5 : Merge  Inputs=4
  NoHwAgDataToSerlCom : Subsystem  TreatAsAtomicUnit=on
  Relational Operator1 : RelationalOperator  RequirementInfo={} %GIDa_71a7d845_40bf_4a37_925d_fd6a479e0667  OutDataTypeStr=boolean
  Relational Operator2 : RelationalOperator  RequirementInfo={} %GIDa_250ba460_efe0_48d9_9422_1dda46894488  OutDataTypeStr=boolean
  Relational Operator4 : RelationalOperator  RequirementInfo={} %GIDa_ed0c9998_f6ad_4f0e_85ab_8891029db1bf  OutDataTypeStr=boolean
  SnsrDataToSerlCom : Subsystem  TreatAsAtomicUnit=on
  SnsrlsDataToSerlCom : Subsystem  TreatAsAtomicUnit=on
  SnsrlsHwAgSeln : Subsystem  TreatAsAtomicUnit=on
  VrfyHwAgCorrln : Subsystem  TreatAsAtomicUnit=on
  SrcSeln : Outport
  HwAgOut : Outport  Port=2
  HwAgConfOut : Outport  Port=3
  HwAgNotCorrd : Outport  Port=4
  HwAgToSerlCom : Outport  Port=5
  HwAgStsToSerlCom : Outport  Port=6
  wires:
  HwAgSnsrls/1 -> [HwAgSnsrls]
  [HwAgCorrdConf] -> VrfyHwAgCorrln/2(HwAgCorrdConf)
  If/2 -> SnsrlsHwAgSeln/Action
  HwAgCorrd/1 -> [HwAgCorrd]
  Merge/1 -> HwAgOut/1
  [HwAgSnsrls] -> ChkCorrln/2(HwAgSnsrls)
  If/1 -> VrfyHwAgCorrln/Action
  [HwAgSnsrls] -> SnsrlsHwAgSeln/1(HwAgSnsrls)
  [HwAgSnsrlsConf] -> SnsrlsHwAgSeln/2(HwAgSnsrlsConf)
  [HwAgCorrd] -> VrfyHwAgCorrln/1(HwAgCorrd)
  HwAg/1 -> VrfyHwAgCorrln/3(HwAg)
  Merge2/1 -> HwAgNotCorrd/1
  Merge3/1 -> SrcSeln/1
  Merge1/1 -> HwAgConfOut/1
  HwAgSnsrlsConf/1 -> [HwAgSnsrlsConf], Relational Operator2/2
  [HwAgCorrdConf] -> Relational Operator1/1
  Constant2/1 -> Relational Operator1/2
  [HwAgSnsrlsConf] -> Relational Operator4/1
  Constant1/1 -> Relational Operator4/2
  Relational Operator4/1 -> If1/2
  Relational Operator2/1 -> If/1
  If1/1 -> ChkCorrln/Action
  [HwAgCorrd] -> ChkCorrln/1(HwAgCorrd)
  Relational Operator1/1 -> If1/1
  VrfyHwAgCorrln/1(HwAgOut) -> Merge/1
  SnsrlsHwAgSeln/1(HwAgOut) -> Merge/2
  VrfyHwAgCorrln/2(HwAgConfOut) -> Merge1/1
  SnsrlsHwAgSeln/2(HwAgConfOut) -> Merge1/2
  VrfyHwAgCorrln/3("HwAgNotCorrd ") -> Merge2/1
  SnsrlsHwAgSeln/3(HwAgNotCorrd) -> Merge2/2
  SnsrlsHwAgSeln/4(SrcSeln) -> Merge3/2
  VrfyHwAgCorrln/4(SrcSeln) -> Merge3/1
  If1/2 -> SnsrDataToSerlCom/Action
  [HwAgCorrd] -> SnsrDataToSerlCom/1(HwAgCorrd)
  [HwAgSnsrls] -> SnsrlsDataToSerlCom/1(HwAgSnsrls)
  If1/3 -> SnsrlsDataToSerlCom/Action
  If1/4 -> NoHwAgDataToSerlCom/Action
  [HwAgCorrdConf] -> ChkCorrln/3(HwAgCorrdConf)
  [HwAgCorrdConf] -> SnsrDataToSerlCom/2(HwAgCorrdConf)
  [HwAgSnsrlsConf] -> SnsrlsDataToSerlCom/2(HwAgSnsrlsConf)
  ChkCorrln/1(HwAgToSerlCom) -> Merge4/1
  SnsrDataToSerlCom/1(HwAgToSerlCom) -> Merge4/2
  SnsrlsDataToSerlCom/1(HwAgToSerlCom) -> Merge4/3
  NoHwAgDataToSerlCom/1(HwAgToSerlCom) -> Merge4/4
  ChkCorrln/2(HwAgStsToSerlCom) -> Merge5/1
  SnsrDataToSerlCom/2(HwAgStsToSerlCom) -> Merge5/2
  SnsrlsDataToSerlCom/2(HwAgStsToSerlCom) -> Merge5/3
  NoHwAgDataToSerlCom/2(HwAgStsToSerlCom) -> Merge5/4
  Merge4/1 -> HwAgToSerlCom/1
  Merge5/1 -> HwAgStsToSerlCom/1
  HwAgCorrdConf/1 -> [HwAgCorrdConf], Relational Operator2/1
